simulink model "ms_inter1"  (Simulink 7.3)
settings: Solver=VariableStepDiscrete  StartTime=0.0  StopTime=10.0  RelTol=1e-3
undefined symbols (not defined in the file or in its folder): my_var
settings Model: Creator=sn00632  LastModifiedBy=sn00632
settings DebuggingCC: SolverPrmCheckMsg=none

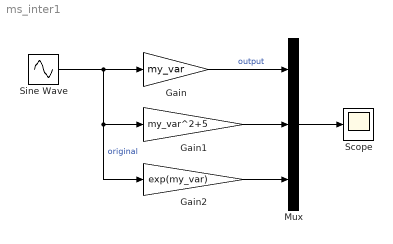
== system ms_inter1 ==
  Gain : Gain  Gain=my_var  ParameterDataType=fixdt(1, 16)  ParameterScaling=2^0  OutDataType=fixdt(1, 16)  OutScaling=2^0
  Gain1 : Gain  Gain=my_var^2+5  ParameterDataType=fixdt(1, 16)  ParameterScaling=2^0  OutDataType=fixdt(1, 16)  OutScaling=2^0
  Gain2 : Gain  Gain=exp(my_var)  ParameterDataType=fixdt(1, 16)  ParameterScaling=2^0  OutDataType=fixdt(1, 16)  OutScaling=2^0
  Mux : Mux  Inputs=3
  Scope : Scope
  Sine Wave : Sin  Amplitude=1  Bias=0  Frequency=1  Phase=0  Samples=10  SampleTime=0  Offset=0
  wires:
  Sine Wave/1 -> Gain/1, Gain1/1, Gain2/1  "original"
  Gain/1 -> Mux/1  "output"
  Gain2/1 -> Mux/3
  Mux/1 -> Scope/1
  Gain1/1 -> Mux/2
